simulink library "csu_eph_spice_lib"  (R2014b)
settings: Solver=ode45  StartTime=0.0  StopTime=10.0  RelTol=1e-3
undefined symbols (not defined in the file or in its folder): csu_grv_mu_earth, csu_grv_mu_sun, pos_m2e_mcmf, pos_m2s_mcmf, spice_time_step_size
libraries: util_quat_lib x2, util_common_lib x2, util_info_lib x1
settings Model: Creator=Bryan Chan  LastModifiedBy=mstewart

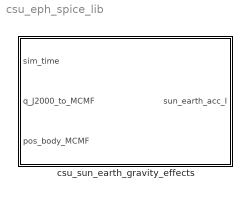
== system csu_eph_spice_lib ==
  csu_sun_earth_gravity_effects : Subsystem

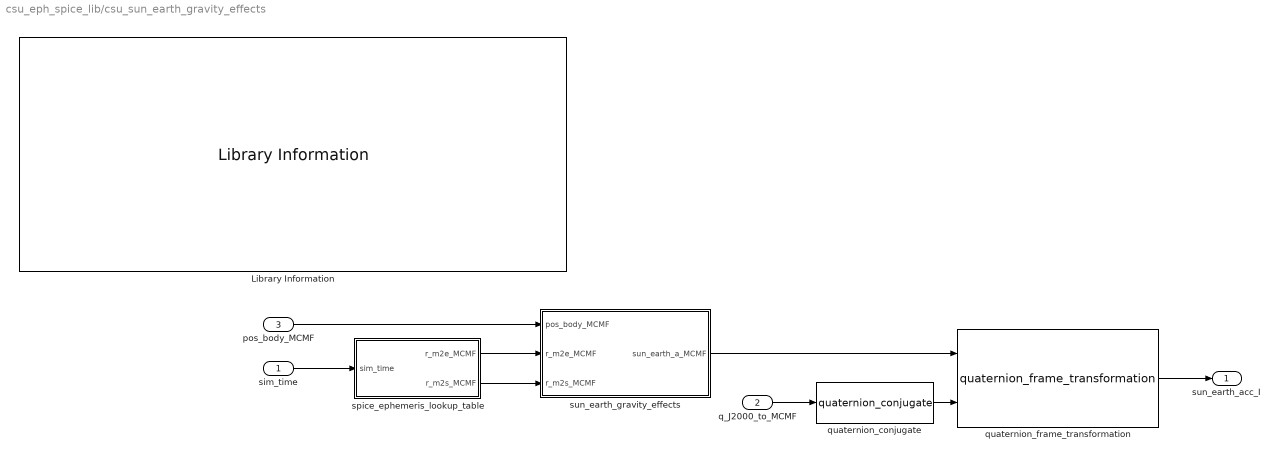
== system csu_eph_spice_lib/csu_sun_earth_gravity_effects ==
  sim_time : Inport
  q_J2000_to_MCMF : Inport  Port=2
  pos_body_MCMF : Inport  Port=3
  Library Information : util_info_lib/Library Information  owner='escrane'
  quaternion_conjugate : util_quat_lib/quaternion_conjugate  SystemSampleTime=-1
  quaternion_frame_transformation : util_quat_lib/quaternion_frame_transformation  SystemSampleTime=-1
  spice_ephemeris_lookup_table : Subsystem
  sun_earth_gravity_effects : Subsystem
  sun_earth_acc_I : Outport
  wires:
  spice_ephemeris_lookup_table/1(r_m2e_MCMF) -> sun_earth_gravity_effects/2(r_m2e_MCMF)
  spice_ephemeris_lookup_table/2(r_m2s_MCMF) -> sun_earth_gravity_effects/3(r_m2s_MCMF)
  q_J2000_to_MCMF/1 -> quaternion_conjugate/1
  quaternion_conjugate/1 -> quaternion_frame_transformation/2
  sun_earth_gravity_effects/1(sun_earth_a_MCMF) -> quaternion_frame_transformation/1
  quaternion_frame_transformation/1 -> sun_earth_acc_I/1
  pos_body_MCMF/1 -> sun_earth_gravity_effects/1(pos_body_MCMF)
  sim_time/1 -> spice_ephemeris_lookup_table/1(sim_time)

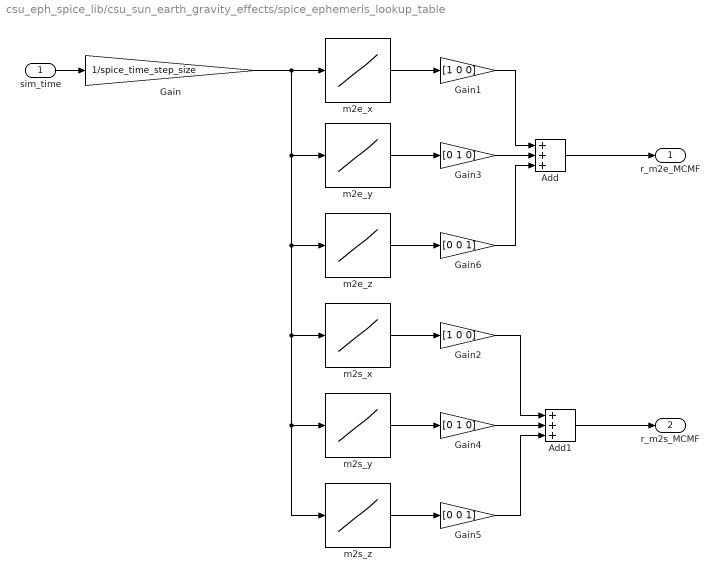
== system csu_eph_spice_lib/csu_sun_earth_gravity_effects/spice_ephemeris_lookup_table ==
  sim_time : Inport
  Add : Sum  Inputs=+++
  Add1 : Sum  Inputs=+++
  Gain : Gain  Gain=1/spice_time_step_size
  Gain1 : Gain  Gain=[1 0 0]
  Gain2 : Gain  Gain=[1 0 0]
  Gain3 : Gain  Gain=[0 1 0]
  Gain4 : Gain  Gain=[0 1 0]
  Gain5 : Gain  Gain=[0 0 1]
  Gain6 : Gain  Gain=[0 0 1]
  m2e_x : Lookup_n-D  NumberOfTableDimensions=1  BreakpointsForDimension1=[1:length(pos_m2e_mcmf)]  Table=pos_m2e_mcmf(:,1)  RndMeth=Simplest  InputSameDT=on
  m2e_y : Lookup_n-D  NumberOfTableDimensions=1  BreakpointsForDimension1=[1:length(pos_m2e_mcmf)]  Table=pos_m2e_mcmf(:,2)  RndMeth=Simplest  InputSameDT=on
  m2e_z : Lookup_n-D  NumberOfTableDimensions=1  BreakpointsForDimension1=[1:length(pos_m2e_mcmf)]  Table=pos_m2e_mcmf(:,3)  RndMeth=Simplest  InputSameDT=on
  m2s_x : Lookup_n-D  NumberOfTableDimensions=1  BreakpointsForDimension1=[1:length(pos_m2s_mcmf)]  Table=pos_m2s_mcmf(:,1)  RndMeth=Simplest  InputSameDT=on
  m2s_y : Lookup_n-D  NumberOfTableDimensions=1  BreakpointsForDimension1=[1:length(pos_m2s_mcmf)]  Table=pos_m2s_mcmf(:,2)  RndMeth=Simplest  InputSameDT=on
  m2s_z : Lookup_n-D  NumberOfTableDimensions=1  BreakpointsForDimension1=[1:length(pos_m2s_mcmf)]  Table=pos_m2s_mcmf(:,3)  RndMeth=Simplest  InputSameDT=on
  r_m2e_MCMF : Outport
  r_m2s_MCMF : Outport  Port=2
  wires:
  sim_time/1 -> Gain/1
  m2e_x/1 -> Gain1/1
  Gain/1 -> m2s_z/1, m2s_y/1, m2s_x/1, m2e_z/1, m2e_y/1, m2e_x/1
  m2e_y/1 -> Gain3/1
  m2e_z/1 -> Gain6/1
  m2s_x/1 -> Gain2/1
  m2s_y/1 -> Gain4/1
  m2s_z/1 -> Gain5/1
  Gain4/1 -> Add1/2
  Gain2/1 -> Add1/1
  Gain5/1 -> Add1/3
  Add1/1 -> r_m2s_MCMF/1
  Gain3/1 -> Add/2
  Gain1/1 -> Add/1
  Gain6/1 -> Add/3
  Add/1 -> r_m2e_MCMF/1

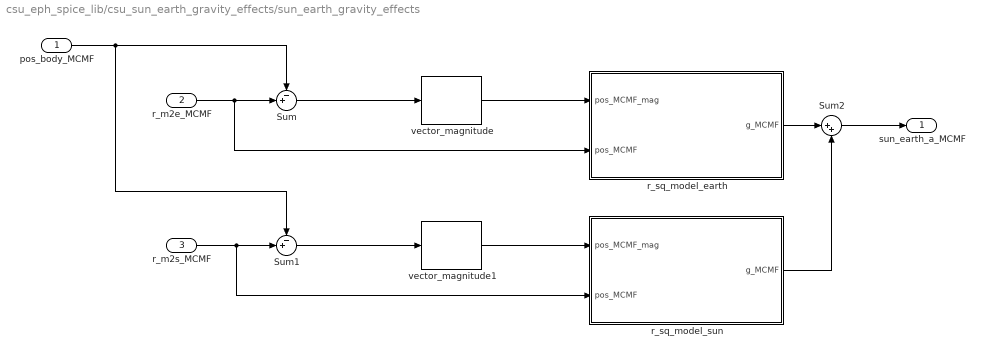
== system csu_eph_spice_lib/csu_sun_earth_gravity_effects/sun_earth_gravity_effects ==
  pos_body_MCMF : Inport
  r_m2e_MCMF : Inport  Port=2
  r_m2s_MCMF : Inport  Port=3
  Sum : Sum  Inputs=-+|
  Sum1 : Sum  Inputs=-+|
  Sum2 : Sum  Inputs=|++
  r_sq_model_earth : Subsystem
  r_sq_model_sun : Subsystem
  vector_magnitude : util_common_lib/vector_magnitude  SystemSampleTime=-1
  vector_magnitude1 : util_common_lib/vector_magnitude  SystemSampleTime=-1
  sun_earth_a_MCMF : Outport
  wires:
  Sum/1 -> vector_magnitude/1
  Sum1/1 -> vector_magnitude1/1
  r_sq_model_earth/1(g_MCMF) -> Sum2/1
  r_sq_model_sun/1(g_MCMF) -> Sum2/2
  pos_body_MCMF/1 -> Sum1/1, Sum/1
  Sum2/1 -> sun_earth_a_MCMF/1
  vector_magnitude/1 -> r_sq_model_earth/1(pos_MCMF_mag)
  r_m2e_MCMF/1 -> r_sq_model_earth/2(pos_MCMF), Sum/2
  r_m2s_MCMF/1 -> r_sq_model_sun/2(pos_MCMF), Sum1/2
  vector_magnitude1/1 -> r_sq_model_sun/1(pos_MCMF_mag)

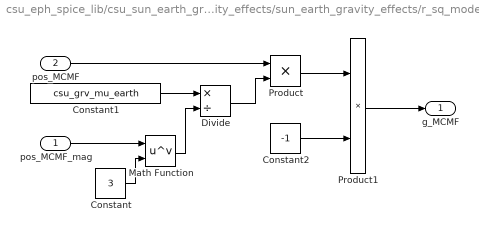
== system csu_eph_spice_lib/csu_sun_earth_gravity_effects/sun_earth_gravity_effects/r_sq_model_earth ==
  pos_MCMF_mag : Inport
  pos_MCMF : Inport  Port=2
  Constant : Constant  Value=3
  Constant1 : Constant  Value=csu_grv_mu_earth
  Constant2 : Constant  Value=-1
  Divide : Product  Inputs=*/
  Math Function : Math  Operator=pow  SaturateOnIntegerOverflow=on
  Product : Product
  Product1 : Product
  g_MCMF : Outport
  wires:
  pos_MCMF_mag/1 -> Math Function/1
  Constant2/1 -> Product1/2
  Product1/1 -> g_MCMF/1
  Product/1 -> Product1/1
  pos_MCMF/1 -> Product/1
  Divide/1 -> Product/2
  Math Function/1 -> Divide/2
  Constant1/1 -> Divide/1
  Constant/1 -> Math Function/2

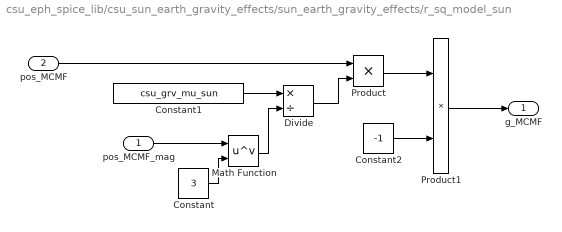
== system csu_eph_spice_lib/csu_sun_earth_gravity_effects/sun_earth_gravity_effects/r_sq_model_sun ==
  pos_MCMF_mag : Inport
  pos_MCMF : Inport  Port=2
  Constant : Constant  Value=3
  Constant1 : Constant  Value=csu_grv_mu_sun
  Constant2 : Constant  Value=-1
  Divide : Product  Inputs=*/
  Math Function : Math  Operator=pow  SaturateOnIntegerOverflow=on
  Product : Product
  Product1 : Product
  g_MCMF : Outport
  wires:
  Constant/1 -> Math Function/2
  Constant1/1 -> Divide/1
  Math Function/1 -> Divide/2
  Divide/1 -> Product/2
  pos_MCMF/1 -> Product/1
  Product/1 -> Product1/1
  Product1/1 -> g_MCMF/1
  Constant2/1 -> Product1/2
  pos_MCMF_mag/1 -> Math Function/1
